simulink model "sf_server"  (Simulink 6.0)
settings: Solver=ode45  StartTime=0.0  StopTime=inf  RelTol=1e-3
PreLoadFcn:
  | queueLength = 10;
CloseFcn:
  | delete(findall(0, 'type', 'figure', 'tag', 'SF_SERVER'))
  | clear('queueLength')
settings Model: CovMetricSettings=dcmtr  Creator=The MathWorks Inc.  LastModifiedBy=batserve  ExtModeAutoUpdateStatusClock=off
settings DataIOCC: SignalLoggingName=logsOut
settings DebuggingCC: CheckExecutionContextPreStartOutputMsg=on  CheckExecutionContextRuntimeOutputMsg=on  SolverPrmCheckMsg=none
settings HardwareCC: TargetUnknown=on

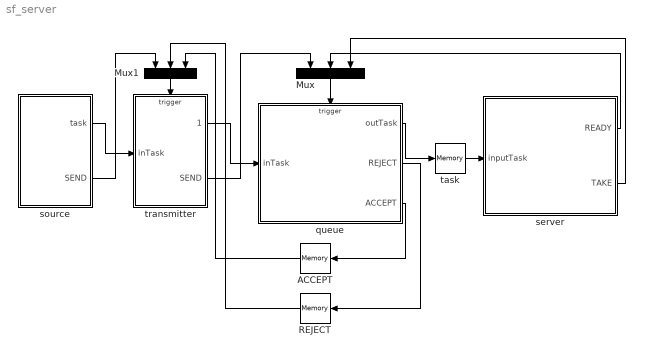
== system sf_server ==
  ACCEPT : Memory  Orientation=left
  Mux : Mux  Orientation=down  Inputs=3
  Mux1 : Mux  Orientation=down  Inputs=3
  REJECT : Memory  Orientation=left
  queue : Stateflow chart  PropExecContextAcrossSSBoundary=on
  server : Stateflow chart  PropExecContextAcrossSSBoundary=on
  source : Stateflow chart  PropExecContextAcrossSSBoundary=on
  task : Memory
  transmitter : Stateflow chart  PropExecContextAcrossSSBoundary=on
  wires:
  queue/1(outTask) -> task/1
  transmitter/1(outTask) -> queue/1(inTask)
  transmitter/2(SEND) -> Mux/1
  server/1(READY) -> Mux/2
  Mux/1 -> queue/Trigger
  server/2(TAKE) -> Mux/3
  source/1(task) -> transmitter/1(inTask)
  source/2(SEND) -> Mux1/1
  Mux1/1 -> transmitter/Trigger
  queue/2(REJECT) -> REJECT/1
  task/1 -> server/1(inputTask)
  REJECT/1 -> Mux1/2
  queue/3(ACCEPT) -> ACCEPT/1
  ACCEPT/1 -> Mux1/3

== stateflow chart queue ==
  state Queue [group]
    state b = is_empty() [function]
      (default) -> (junction 11) : {b = front == back && !incremented;}
    state enqueue(d) [function]
      (default) -> (junction 13)
      (junction 13) -> (junction 14) : [is_full()]
          | {ml.error('Queue overflow');}
      (junction 13) -> (junction 15) : {back = increment(back);
          | incremented = 1;
          | data[back] = d;
          | set_queue(data, front, back, is_full());}
    state d = dequeue() [function]
      (default) -> (junction 16)
      (junction 16) -> (junction 17) : [is_empty()]
          | {ml.error('Queue underflow');}
      (junction 16) -> (junction 20) : {front = increment(front);
          | incremented = 0;
          | d = data[front];
          | set_queue(data, front, back, 0);}
    state next = increment(i) [function]
      (junction 18) -> (junction 12) : [next > queueLength]
          | {next = 1;}
      (default) -> (junction 18) : {next = i+1;}
    state b = is_full() [function]
      (default) -> (junction 19) : {b = front == back && incremented;}
  (default) -> (junction 10) : ENQUEUE
  (default) -> (junction 21) : CLEAR
      | {outTask = 0;}
  (junction 10) -> (junction 22) : [Queue.is_full()]
      | {REJECT;}
  (junction 10) -> (junction 23) : {ACCEPT;
      | Queue.enqueue(inTask);}
  (junction 26) -> (junction 24) : {outTask = Queue.dequeue();}
  (junction 26) -> (junction 25) : [Queue.is_empty()]
      | {outTask = 0;}
  (default) -> (junction 26) : DEQUEUE
  data: data local double size=queueLength; front local double size=1; back local double size=1; incremented local boolean size=1; b function_output boolean size=1; d function_input int32 size=1; d function_output int32 size=1; next function_output int32 size=1; i function_input int32 size=1; b function_output boolean size=1; queue function_input double size=queueLength; front function_input double size=1; back function_input double size=1; isFull function_input double size=1; inTask input double size=1; outTask output double size=1
  events: ENQUEUE input EITHER_EDGE_EVENT; DEQUEUE input EITHER_EDGE_EVENT; CLEAR input EITHER_EDGE_EVENT; REJECT output EITHER_EDGE_EVENT; ACCEPT output EITHER_EDGE_EVENT
  function set_queue(queue,front,back,isFull):
    | function set_queue(queue, front, back, isFull)
    | 
    |     for i = queueLength:-1:1
    |         string = ' ';
    | 
    |         if front ~= back || isFull
    |             front = increment(front);
    |             string = int2str(queue(front));
    |             isFull = 0;
    |         end
    | 
    |         set(queueText(i), 'String', string);
    |     end
    | 
    | function i = increment(i)
    |     i = i + 1;
    |     if i > queueLength
    |         i = 1;
    |     end

== stateflow chart server ==
  state Idle
    READY;
  state Busy
  Idle -> Busy : [inputTask]
      | {taskTime = 2*inputTask;
      | TAKE;
      | process_task(inputTask);}
  Busy -> Idle : [after(taskTime, tick)]
      | {process_task(0);}
  (default) -> Idle
  Idle -> Idle
  data: task function_input double size=1; inputTask input double size=1; taskTime local double size=1
  events: READY output EITHER_EDGE_EVENT; TAKE output EITHER_EDGE_EVENT
  function process_task(task):
    | function process_task(task)
    | 
    | string = ' ';
    | 
    | if task
    |     string = int2str(task);
    | end
    | 
    | set(processText, 'String', string);

== stateflow chart transmitter ==
  (default) -> (junction 85) : TRANSMIT
      | {send_task(inTask);
      | outTask = inTask;
      | SEND;}
  (default) -> (junction 86) : REJECT
      | {reject_task();}
  (default) -> (junction 87) : ACCEPT
      | {accept_task();}
  data: task function_input double size=1; outTask output double size=1; inTask input double size=1
  events: SEND output EITHER_EDGE_EVENT; TRANSMIT input EITHER_EDGE_EVENT; REJECT input EITHER_EDGE_EVENT; ACCEPT input EITHER_EDGE_EVENT
  function init_gui:
    | function init_gui
    | 
    | if ~fig
    |     % see if there is an existing figure
    |     figTemp = findall(0, 'type', 'figure', 'tag', 'SF_SERVER');
    |     if ~isempty(figTemp)
    |         deleteFig = 0;
    |         fig = figTemp;
    |         lastObj = fig;
    |         sendText = get(lastObj, 'UserData');
    |         lastObj = sendText;
    |         for i = 1:queueLength
    |             queueText(i) = get(lastObj, 'UserData');
    |             if ~queueText(i)
    |                 deleteFig = 1;
    |                 break;
    |             end
    |             set(queueText(i), 'String', '');
    |             lastObj = queueText(i);
    |         end
    |         if ~deleteFig
    |             processText = get(lastObj, 'UserData');
    |             if ~processText
    |                 deleteFig = 1;
    |             else
    |                 deleteFig = get(processText, 'UserData')
    |             end
    |         end
    |         if deleteFig
    |             delete(fig);
    |             fig = 0;
    |         end
    |     end
    | end
    | 
    | if ~fig
    |     % screen size etiqette
    |     units = 'points';
    |     screenUnits = get(0, 'Units');
    |     set(0, 'Units', units);
    |     screenSize = zeros(1,4);
    |     screenSize = get(0, 'ScreenSize');
    |     set(0, 'Units', screenUnits);
    |     
    |     backgroundColor = get(0, 'DefaultUIControlBackgroundColor');
    | 
    |     fontSize = 48;
    |     buffer = 10;
    |     textWidth = 35;    
    |     textY = 50;
    |     rectHeight = 60;
    |     rectWidth = textWidth-5;
    |     rectY = textY - rectHeight/2;
    | 
    |     
    |     % default figure size
    |     figureHeight = 2*textY;
    |     figureWidth = 4*buffer+(queueLength+2)*textWidth;
    | 
    |     % make sure the initial size is less than 90% of the screen in either direction
    |     figureWidth = min(figureWidth, .9*screenSize(3));
    |     figureHeight = min(figureHeight, .9*screenSize(4));
    | 
    |     % create a figure
    |     fig = figure('doubleBuffer', 'on',...
    |                  'MenuBar', 'none',...
    |                  'Name', 'Server Display',...
    |                  'Tag', 'SF_SERVER',...
    |                  'NumberTitle', 'off',...
    |                  'HandleVisibility', 'off',...
    |                  'IntegerHandle', 'off',...
    |                  'Color', backgroundColor,...
    |                  'Units', units,...
    |                  'DefaultUIControlUnits', units,...
    |                  'Position', [(screenSize(3)-figureWidth)/2 (screenSize(4)-figureHeight)/2 figureWidth figureHeight]);
    | 
    |     lastObj = fig;
    |     
    |     figAxes = axes('Parent', fig,...
    |                    'Visible', 'off',...
    |                    'Position', [0 0 1 1],...
    |                    'XLim', [0 figureWidth],...
    |                    'YLim', [0 figureHeight]);
    | 
    |     sendText = text(buffer, textY, '',...
    |                     'Parent', figAxes,...
    |                     'Color', 'blue',...
    |                     'BackgroundColor', backgroundColor,...
    |                     'FontSize', fontSize);
    | 
    |     set(lastObj, 'UserData', sendText);
    |     lastObj = sendText;
    |     
    |     for i = 1:queueLength
    |         rectangle('Position', [2*buffer+i*textWidth-2, rectY, rectWidth, rectHeight],...
    |                   'FaceColor', 'black',...
    |                   'EdgeColor', 'none',...
    |                   'Parent', figAxes);
    |         queueText(i) = text(2*buffer+i*textWidth, textY, '',...
    |                             'Parent', figAxes,...
    |                             'Color', 'green',...
    |                             'BackgroundColor', 'black',...
    |                             'FontSize', fontSize);
    |         set(lastObj, 'UserData', queueText(i));
    |         lastObj = queueText(i);
    |     end
    |    
    |     processText = text(3*buffer+(queueLength+1)*textWidth, textY, '',...
    |                        'Parent', figAxes,...
    |                        'Color', 'black',...
    |                        'BackgroundColor', backgroundColor,...
    |                        'FontSize', fontSize,...
    |                        'UserData', 0);
    | 
    |     set(lastObj, 'UserData', processText);
    | end
  function send_task(task):
    | function send_task(task)
    | 
    | if ~fig
    |     init_gui;
    | end
    | 
    | set(sendText, 'String', int2str(task), 'Color', 'blue');
  function reject_task():
    | function reject_task
    | 
    | set(sendText, 'Color', 'red');
  function accept_task():
    | function accept_task
    | 
    | set(sendText, 'String', '');

== stateflow chart source ==
  state Pause
    ex: ml.pause(.1);
  state Send
  Send -> (junction 102) : {x = ml.floor(ml.rand()*20);}
  (junction 102) -> (junction 103) : [x>=19]{task = 5;}
  (junction 102) -> (junction 104)
  (junction 104) -> (junction 105) : [x>=18]{task = 4;}
  (junction 104) -> (junction 106)
  (junction 106) -> (junction 107) : [x>=17]{task = 3;}
  (junction 106) -> (junction 108)
  (junction 108) -> (junction 109) : [x>=15]{task = 2;}
  (junction 108) -> (junction 110)
  (junction 110) -> (junction 111) : [x>=14]{task = 1;}
  (junction 103) -> (junction 105)
  (junction 105) -> (junction 107)
  (junction 107) -> (junction 109)
  (junction 109) -> (junction 111)
  (junction 111) -> (junction 112) : {SEND;}
  (junction 110) -> (junction 113)
  (default) -> Send
  (junction 113) -> (junction 112)
  Pause -> Send
  (junction 112) -> (junction 114)
  (junction 114) -> Pause
  data: x local double size=1; task output double size=1
  events: SEND output EITHER_EDGE_EVENT
